simulink library "Auto_transformer_Starter"  (R2024a)
settings: Solver=VariableStepAuto  StartTime=0.0  StopTime=10.0  RelTol=1e-3
libraries: spsThreePhaseBreakerLib x3, spsVariableRatioTransformerLib x3, spsGroundLib x2, simulink_extras x1, spsVoltageMeasurementLib x1
settings Model: Creator=gshma  LastModifiedBy=gshma

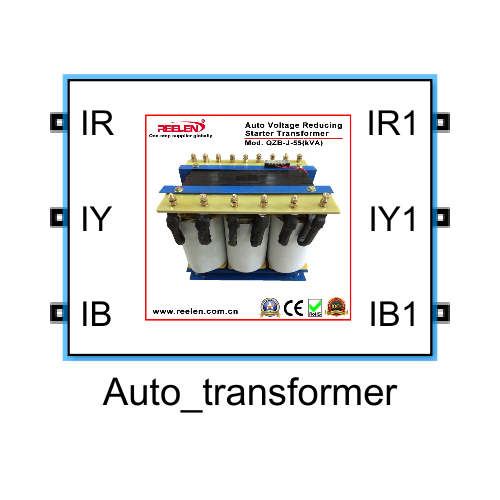
[thumbnail: Simulink's stored preview of the top-level diagram]
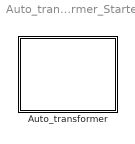
== system Auto_transformer_Starter ==
  Auto_transformer : Subsystem
      mask Display: image('autotaren.webp', [0,0,0,0,75,75]);

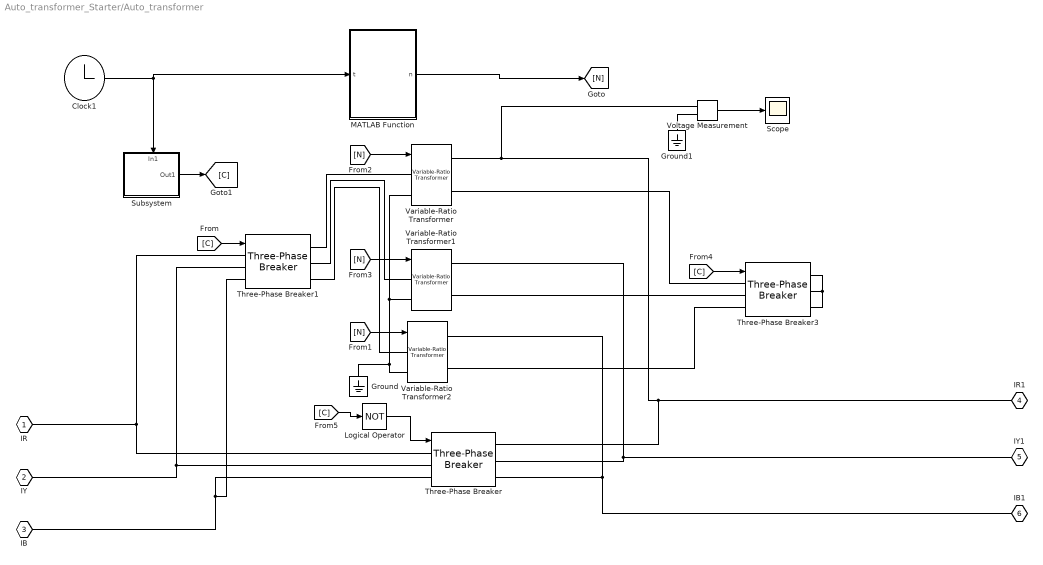
== system Auto_transformer_Starter/Auto_transformer ==
  Clock1 : Clock
      settings: Decimation=1000
  Ground : spsGroundLib/Ground  LConnTagsString=a
  Ground1 : spsGroundLib/Ground  LConnTagsString=a
  Logical Operator : Logic  Operator=NOT  AllPortsSameDT=off  OutDataTypeStr=boolean
  MATLAB Function : MATLAB Function  TreatAsAtomicUnit=on
  Scope : Scope
  Subsystem : Subsystem
      settings: PortSchema="{\"entries\":[{\"content\":{\"sides\":[{\"content\":{},\"type\":\"ConnectorPlacement.EquallySpacedRectSide\",\"uuid\":\"eeea18b9-380b-488c-afba-283aabc25f85\"},{\"content\":{\"connectorIds\":[\"Out1\"],\"side\":\"RIGHT\"},\"type\":\"ConnectorPlacement.EquallySpacedRectSide\",\"uuid\":\"b5cdad00-14f9-426f-8cac-c80f210bc817\"},{\"content\":{\"connectorIds\":[\"In1\"],\"side\":\"TOP\"},\"type\":\"ConnectorPlacement.EquallySpacedRectSide\",\"uuid\":\"d8660c5f-ab56-4d32-b432-a9ce1bc682f2\"}]},\"type\":\"ConnectorPlacement.EquallySpacedConnector\",\"uuid\":\"80a26fe6-a8a6-4d75-a5f0-c797e7c8950d\"}],\"packageUris\":[\"http://schema.mathworks.com/mf0/Connector/R2020b\"],\"version\":\"1.0\"}"
      mask Display: image('microcontroller.jpeg');
  Three-Phase Breaker : spsThreePhaseBreakerLib/Three-Phase Breaker  InitialState=open  SwitchA=on  SwitchB=on  SwitchC=on  SwitchTimes="[1/60  5/60]"  External=on  BreakerResistance=0.01  SnubberResistance=1e6  SnubberCapacitance=inf  Measurements=None
  Three-Phase Breaker1 : spsThreePhaseBreakerLib/Three-Phase Breaker  InitialState=closed  SwitchA=on  SwitchB=on  SwitchC=on  SwitchTimes="[1/60  5/60]"  External=on  BreakerResistance=0.01  SnubberResistance=1e6  SnubberCapacitance=inf  Measurements=None
  Three-Phase Breaker3 : spsThreePhaseBreakerLib/Three-Phase Breaker  InitialState=closed  SwitchA=on  SwitchB=on  SwitchC=on  SwitchTimes="[1/60  5/60]"  External=on  BreakerResistance=0.01  SnubberResistance=1e6  SnubberCapacitance=inf  Measurements=None
  Variable-Ratio Transformer : spsVariableRatioTransformerLib/Variable-Ratio Transformer
      settings: LibrarySourceBlock=|
      | sps_lib/Passives/Variable-Ratio
      | Transformer
  Variable-Ratio Transformer1 : spsVariableRatioTransformerLib/Variable-Ratio Transformer
      settings: LibrarySourceBlock=|
      | sps_lib/Passives/Variable-Ratio
      | Transformer
  Variable-Ratio Transformer2 : spsVariableRatioTransformerLib/Variable-Ratio Transformer
      settings: LibrarySourceBlock=|
      | sps_lib/Passives/Variable-Ratio
      | Transformer
  Voltage Measurement : spsVoltageMeasurementLib/Voltage Measurement  PhasorSimulation=off  OutputType=Complex  PSBequivalent=0
  IR : PMIOPort  Tag=simrfV2util1/Connection Port  Side=Left
  IY : PMIOPort  Tag=simrfV2util1/Connection Port  Port=2  Side=Left
  IB : PMIOPort  Tag=simrfV2util1/Connection Port  Port=3  Side=Left
  IR1 : PMIOPort  Tag=simrfV2util1/Connection Port  Port=4  Side=Right
  IY1 : PMIOPort  Tag=simrfV2util1/Connection Port  Port=5  Side=Right
  IB1 : PMIOPort  Tag=simrfV2util1/Connection Port  Port=6  Side=Right
  wires:
  [N] -> Variable-Ratio Transformer1/1
  Logical Operator/1 -> Three-Phase Breaker/1
  [C] -> Three-Phase Breaker1/1
  [C] -> Logical Operator/1
  MATLAB Function/1(n) -> [N]
  [C] -> Three-Phase Breaker3/1
  [N] -> Variable-Ratio Transformer2/1
  Subsystem/1(Out1) -> [C]
  Voltage Measurement/1 -> Scope/1
  [N] -> Variable-Ratio Transformer/1
  Clock1/1 -> MATLAB Function/1(t), Subsystem/1(In1)
  connections:
  Variable-Ratio Transformer2/LConn2 -- Variable-Ratio Transformer/LConn2 -- Variable-Ratio Transformer1/LConn2 -- Ground/LConn1
  IB1/RConn1 -- Variable-Ratio Transformer2/RConn1 -- Three-Phase Breaker/RConn3
  Three-Phase Breaker1/LConn3 -- Three-Phase Breaker/LConn3 -- IB/RConn1
  Three-Phase Breaker/LConn1 -- IR/RConn1 -- Three-Phase Breaker1/LConn1
  Three-Phase Breaker/RConn2 -- Variable-Ratio Transformer1/RConn1 -- IY1/RConn1
  IR1/RConn1 -- Variable-Ratio Transformer/RConn1 -- Voltage Measurement/LConn1 -- Three-Phase Breaker/RConn1
  Three-Phase Breaker3/RConn2 -- Three-Phase Breaker3/RConn1 -- Three-Phase Breaker3/RConn3
  Three-Phase Breaker/LConn2 -- IY/RConn1 -- Three-Phase Breaker1/LConn2
  Ground1/LConn1 -- Voltage Measurement/LConn2
  Three-Phase Breaker1/RConn2 -- Variable-Ratio Transformer1/LConn1
  Three-Phase Breaker1/RConn1 -- Variable-Ratio Transformer/LConn1
  Three-Phase Breaker3/LConn1 -- Variable-Ratio Transformer/RConn2
  Three-Phase Breaker1/RConn3 -- Variable-Ratio Transformer2/LConn1
  Three-Phase Breaker3/LConn3 -- Variable-Ratio Transformer2/RConn2
  Three-Phase Breaker3/LConn2 -- Variable-Ratio Transformer1/RConn2

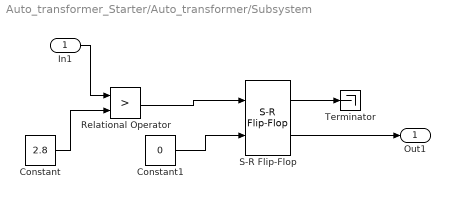
== system Auto_transformer_Starter/Auto_transformer/Subsystem ==
  In1 : Inport
  Constant : Constant  Value=2.8  SampleTime=0.001
  Constant1 : Constant  Value=0  OutDataTypeStr=boolean  SampleTime=0.0001
  Relational Operator : RelationalOperator  Operator=>  OutDataTypeStr=boolean  RndMeth=Simplest  InputSameDT=off
  S-R Flip-Flop : simulink_extras/Flip Flops/S-R Flip-Flop  initial_condition=0
  Terminator : Terminator
  Out1 : Outport
  wires:
  S-R Flip-Flop/1 -> Terminator/1
  In1/1 -> Relational Operator/1
  Constant/1 -> Relational Operator/2
  Constant1/1 -> S-R Flip-Flop/2
  Relational Operator/1 -> S-R Flip-Flop/1
  S-R Flip-Flop/2 -> Out1/1

== matlab function Auto_transformer_Starter/Auto_transformer/MATLAB Function ==
  data: t input; n output
function n = Control_logic(t)
    if t >= 0 && t < 0.5
        n = 0.55;  % Voltage ratio at 50%
    elseif t >=0.5 && t < 1
        n = 0.65;  % Voltage ratio at 65%
    elseif t >=1 && t < 1.4
        n = 0.75;  % Voltage ratio at 65%
    elseif t >=1.4 && t < 1.9
        n = 0.85;  % Voltage ratio at 65%
    elseif t >=1.9 && t < 2.2
        n = 0.95;
    else
        n = 1;  % Voltage ratio at 80%
    end
end
